simulink model "RC_3L_PWM"  (R2013b)
settings: Solver=FixedStepDiscrete  SolverMode=SingleTasking  StartTime=0.0  StopTime=1  FixedStep=Tpas  RelTol=1e-3
undefined symbols (not defined in the file): ASF3, Cbus, DAFE, fmod4Q, Freq, IAFE3L, Iv, Kac, Lac, NAFE, PAFE3L, Pv, Rac, Rch, Satv, Tpas, Vac, Vdc
libraries: powerlib x39, simulink x22, powerlib_meascontrol x16
settings Model: Creator=LiberT  LastModifiedBy=LiberT
settings DataIOCC: SignalLoggingSaveFormat=ModelDataLogs
settings OptimizationCC: ExpressionDepthLimit=2147483647
settings DebuggingCC: MultiTaskDSMMsg=warning  MultiTaskCondExecSysMsg=none  FcnCallInpInsideContextMsg=EnableAllAsWarning  StateNameClashWarn=warning
settings RTWCC: IncludeERTFirstTime=on

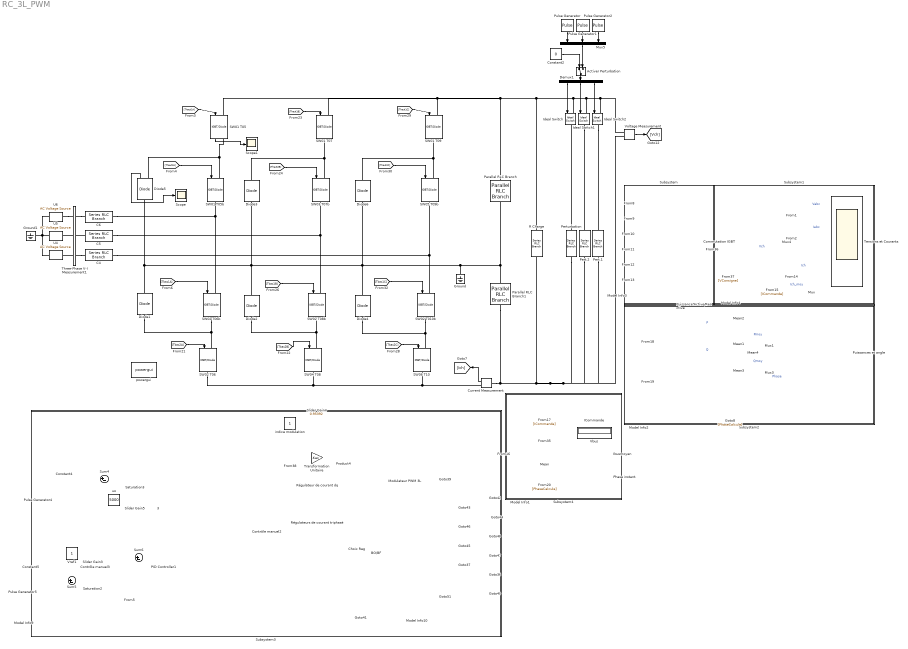
== system RC_3L_PWM ==
  " 3" : ManualSwitch
  Activer Perturbation : ManualSwitch
  BO/BF : ManualSwitch  CurrentSetting=0
  C4 : powerlib/Elements/Series RLC Branch  LConnTagsString=__new0  RConnTagsString=__new0  BranchType=L  Resistance=Rac  Inductance=Lac  SetiL0=off  InitialCurrent=0  Capacitance=300e-3  Setx0=off  InitialVoltage=0  Measurements=None
  C5 : powerlib/Elements/Series RLC Branch  LConnTagsString=__new0  RConnTagsString=__new0  BranchType=L  Resistance=Rac  Inductance=Lac  SetiL0=off  InitialCurrent=0  Capacitance=300e-3  Setx0=off  InitialVoltage=0  Measurements=None
  C6 : powerlib/Elements/Series RLC Branch  LConnTagsString=__new0  RConnTagsString=__new0  BranchType=L  Resistance=Rac  Inductance=Lac  SetiL0=off  InitialCurrent=0  Capacitance=300e-3  Setx0=off  InitialVoltage=0  Measurements=None
  Choix Reg : ManualSwitch  CurrentSetting=0
  Commutation IGBT : Scope  NumInputPorts=6
      settings: TickLabels=on  TimeRange=0.002  YMin=-0.2~-0.2~-0.2~-0.2~-0.2~-0.2  YMax=1.2~1.2~1.2~1.2~1.2~1.2
  Constant2 : Constant  Value=0
  Constant4 : Constant  Value=6000
  Constant5 : Constant  Value=6000
  Contrôle manuel2 : ManualSwitch  CurrentSetting=0
  Contrôle manuel3 : ManualSwitch
  Current Measurement : powerlib/Measurements/Current Measurement  PhasorSimulation=off  OutputType=Complex  PSBequivalent=0
  Demux1 : Demux  Outputs=3
  Diode{1..4,6} (5 alike) : powerlib/Power Electronics/Diode  Ron=0.001  Lon=0  Vf=0.8  IC=0  UseSnubber=off  Rs=500  Cs=inf  Measurements=off
  Diode5 : powerlib/Power Electronics/Diode  Ron=0.001  Lon=0  Vf=0.8  IC=0  UseSnubber=off  Rs=500  Cs=inf  Measurements=on
  Ground : powerlib/Elements/Ground  LConnTagsString=a
  Ground1 : powerlib/Elements/Ground  LConnTagsString=a
  "ICommande " : Display
  Ibusmoyen : Display
  Ideal Switch : powerlib/Power Electronics/Ideal Switch  Ron=0.001  Lon=0  IC=0  Rs=1e5  Cs=inf  Measurements=off
  Ideal Switch1 : powerlib/Power Electronics/Ideal Switch  Ron=0.001  Lon=0  IC=0  Rs=1e5  Cs=inf  Measurements=off
  Ideal Switch2 : powerlib/Power Electronics/Ideal Switch  Ron=0.001  Lon=0  IC=0  Rs=1e5  Cs=inf  Measurements=off
  Mean : powerlib_meascontrol/Measurements/Mean  Freq=50  Vinit=0  Ts=Tpas
  Mean1 : powerlib_meascontrol/Measurements/Mean  Freq=50  Vinit=0  Ts=Tpas
  Mean2 : powerlib_meascontrol/Measurements/Mean  Freq=fmod4Q  Vinit=0  Ts=Tpas
  Mean3 : powerlib_meascontrol/Measurements/Mean  Freq=50  Vinit=0  Ts=Tpas
  Mean4 : powerlib_meascontrol/Measurements/Mean  Freq=fmod4Q  Vinit=0  Ts=Tpas
  Model Info{1..4} (4 alike) : simulink/Model-Wide Utilities/Model Info  InitialBlockCM=None  BlockCM=None  Frame=on  DisplayStringWithTags=Résultats  HorizontalTextAlignment=Center  LeftAlignmentValue=0.5  SourceBlockDiagram=RC_3L_PWM  TagMaxNumber=20
  Model Info10 : simulink/Model-Wide Utilities/Model Info  InitialBlockCM=None  BlockCM=None  Frame=on  DisplayStringWithTags=Commande onduleur NPC3L  HorizontalTextAlignment=Center  LeftAlignmentValue=0.5  SourceBlockDiagram=RC_3L_PWM  TagMaxNumber=20
  Model Info9 : simulink/Model-Wide Utilities/Model Info  InitialBlockCM=None  BlockCM=None  Frame=on  DisplayStringWithTags=Commande AFE  HorizontalTextAlignment=Center  LeftAlignmentValue=0.5  SourceBlockDiagram=RC_3L_PWM  TagMaxNumber=20
  Modulateur PWM 3L : Subsystem
  Mux{,1,3..4} (4 alike) : Mux  Inputs=2
  Mux5 : Mux  Inputs=3
  PID Controller1 : simulink/Continuous/PID Controller  Controller=PI  TimeDomain=Discrete-time  SampleTime=Tpas  IntegratorMethod=Forward Euler  FilterMethod=Forward Euler  Form=Parallel  P=Pv  I=Iv  D=0  N=100  InitialConditionSource=internal  InitialConditionForIntegrator=0  InitialConditionForFilter=0  ExternalReset=none  LimitOutput=on  UpperSaturationLimit=Satv  LowerSaturationLimit=-Satv  LinearizeAsGain=on  AntiWindupMode=clamping  Kb=1  TrackingMode=off  Kt=1  PParamMin=[]  PParamMax=[]  IParamMin=[]  IParamMax=[]  DParamMin=[]  DParamMax=[]  NParamMin=[]  NParamMax=[]  KbParamMin=[]  KbParamMax=[]  KtParamMin=[]  KtParamMax=[]  POutMin=[]  POutMax=[]  IOutMin=[]  IOutMax=[]  DOutMin=[]  DOutMax=[]  NOutMin=[]  NOutMax=[]  KbOutMin=[]  KbOutMax=[]  KtOutMin=[]  KtOutMax=[]  IntegratorOutMin=[]  IntegratorOutMax=[]  FilterOutMin=[]  FilterOutMax=[]  SumOutMin=[]  SumOutMax=[]  SumI1OutMin=[]  SumI1OutMax=[]  SumI2OutMin=[]  SumI2OutMax=[]  SumI3OutMin=[]  SumI3OutMax=[]  SumDOutMin=[]  SumDOutMax=[]  SaturationOutMin=[]  SaturationOutMax=[]  IntegratorContinuousStateAttributes=''  IntegratorStateMustResolveToSignalObject=off  IntegratorRTWStateStorageClass=Auto  FilterContinuousStateAttributes=''  FilterStateMustResolveToSignalObject=off  FilterRTWStateStorageClass=Auto
  Parallel RLC Branch : powerlib/Elements/Parallel RLC Branch  LConnTagsString=a  RConnTagsString=__new0  BranchType=C  Resistance=9.26  Inductance=1e-3  SetiL0=off  InitialCurrent=0  Capacitance=Cbus*2  Setx0=on  InitialVoltage=Vdc/2  Measurements=None
  Parallel RLC Branch1 : powerlib/Elements/Parallel RLC Branch  LConnTagsString=a  RConnTagsString=__new0  BranchType=C  Resistance=9.26  Inductance=1e-3  SetiL0=off  InitialCurrent=0  Capacitance=Cbus*2  Setx0=on  InitialVoltage=Vdc/2  Measurements=None
  Pert.1 : powerlib/Elements/Series RLC Branch  LConnTagsString=__new0  RConnTagsString=__new0  BranchType=R  Resistance=50  Inductance=0  SetiL0=off  InitialCurrent=0  Capacitance=inf  Setx0=off  InitialVoltage=0  Measurements=None
  Pert.2 : powerlib/Elements/Series RLC Branch  LConnTagsString=__new0  RConnTagsString=__new0  BranchType=R  Resistance=50  Inductance=0  SetiL0=off  InitialCurrent=0  Capacitance=inf  Setx0=off  InitialVoltage=0  Measurements=None
  Perturbation : powerlib/Elements/Series RLC Branch  LConnTagsString=__new0  RConnTagsString=__new0  BranchType=R  Resistance=50  Inductance=0  SetiL0=off  InitialCurrent=0  Capacitance=inf  Setx0=off  InitialVoltage=0  Measurements=None
  Phase instant. : Display
  Product4 : Product
  Puissance Active/Reactive : Subsystem
  Puissances et angle : Scope  NumInputPorts=3
      settings: TickLabels=on  TimeRange=0.04  YMin=-5.5e+06~-500000~-120  YMax=500000~250000~50  SaveName=ScopeData2
  Pulse Generator : DiscretePulseGenerator  Period=floor((1/Tpas)/2)  PulseWidth=floor((1/Tpas)/4)  SampleTime=Tpas
  Pulse Generator1 : DiscretePulseGenerator  Period=floor((1/Tpas)/3)  PulseWidth=floor((1/Tpas)/6)  SampleTime=Tpas
  Pulse Generator2 : DiscretePulseGenerator  Period=floor((1/Tpas))  PulseWidth=floor((1/Tpas)/2)  SampleTime=Tpas
  Pulse Generator4 : DiscretePulseGenerator  Amplitude=12000  Period=floor(.4/Tpas)  PulseWidth=floor(.4/2/Tpas)  SampleTime=Tpas
  Pulse Generator5 : DiscretePulseGenerator  Amplitude=12000  Period=floor(.2/Tpas)  PulseWidth=floor(.2/2/Tpas)  SampleTime=Tpas
  R Charge : powerlib/Elements/Series RLC Branch  LConnTagsString=__new0  RConnTagsString=__new0  BranchType=R  Resistance=Rch  Inductance=0  SetiL0=off  InitialCurrent=0  Capacitance=inf  Setx0=off  InitialVoltage=0  Measurements=None
  Régulateur de courant dq : Subsystem
  Régulateurs de courant triphasé : Subsystem
  SW01 T05 : powerlib/Power Electronics/IGBT//Diode  Ron=1e-3  Rs=1e5  Cs=Tpas  Measurements=on
  SW01 T05b : powerlib/Power Electronics/IGBT//Diode  Ron=1e-3  Rs=1e5  Cs=Tpas  Measurements=off
  SW01 T07 : powerlib/Power Electronics/IGBT//Diode  Ron=1e-3  Rs=1e5  Cs=Tpas  Measurements=off
  SW01 T09 : powerlib/Power Electronics/IGBT//Diode  Ron=1e-3  Rs=1e5  Cs=Tpas  Measurements=off
  SW02 T010b : powerlib/Power Electronics/IGBT//Diode  Ron=1e-3  Rs=1e5  Cs=Tpas  Measurements=off
  SW02 T06 : powerlib/Power Electronics/IGBT//Diode  Ron=1e-3  Rs=1e5  Cs=Tpas  Measurements=off
  SW02 T06b : powerlib/Power Electronics/IGBT//Diode  Ron=1e-3  Rs=1e5  Cs=Tpas  Measurements=off
  SW02 T08b : powerlib/Power Electronics/IGBT//Diode  Ron=1e-3  Rs=1e5  Cs=Tpas  Measurements=off
  SW03 T07b : powerlib/Power Electronics/IGBT//Diode  Ron=1e-3  Rs=1e5  Cs=Tpas  Measurements=off
  SW04 T08 : powerlib/Power Electronics/IGBT//Diode  Ron=1e-3  Rs=1e5  Cs=Tpas  Measurements=off
  SW05 T09b : powerlib/Power Electronics/IGBT//Diode  Ron=1e-3  Rs=1e5  Cs=Tpas  Measurements=off
  SW06 T10 : powerlib/Power Electronics/IGBT//Diode  Ron=1e-3  Rs=1e5  Cs=Tpas  Measurements=off
  Saturation2 : Saturate  UpperLimit=5500  LowerLimit=4800
  Saturation3 : Saturate  UpperLimit=5000  LowerLimit=1000
  Scope : Scope
      settings: SaveName=DIODE
  Scope1 : Scope
      settings: SaveName=IGBT
  Slider Gain3 : simulink/Math Operations/Slider Gain  low=0  gain=5000  high=7000
  Slider Gain4 : simulink/Math Operations/Slider Gain  low=0  gain=0.95392  high=1
  Slider Gain5 : simulink/Math Operations/Slider Gain  low=0  gain=0  high=1
  Subsystem : Subsystem
      mask Display: disp('')
  Subsystem1 : Subsystem
      mask Display: disp('')
  Subsystem2 : Subsystem
      mask Display: disp('')
  Subsystem3 : Subsystem
      mask Display: disp('')
  Subsystem4 : Subsystem
      mask Display: disp('')
  Sum4 : Sum  Inputs=|+-
  Sum5 : Sum  Inputs=|+-
  Sum6 : Sum  Inputs=|+-
  Tensions et Courants : Scope  NumInputPorts=4
      settings: TickLabels=on  ShowLegends=on  TimeRange=0.4  YMin=-2000~-2000~5010~-2000  YMax=2000~2000~5100~2000  SaveName=AFE3LEVEL  MaxDataPoints=50000
  Three-Phase V-I Measurement1 : powerlib/Measurements/Three-Phase V-I Measurement  VoltageMeasurement=phase-to-ground  SetLabelV=on  LabelV=Vabc  Vpu=off  VpuLL=off  CurrentMeasurement=yes  SetLabelI=on  LabelI=Iabc  Ipu=off  Pbase=100e6  Vbase=500e3  OutputType=Complex  PhasorSimulation=off  PSBequivalent=0
  Transformation Unitaire : Gain  Gain=-Kac
  U4 : powerlib/Electrical Sources/AC Voltage Source  Amplitude=Vac*sqrt(2/3)  Phase=120  Frequency=Freq  SampleTime=Tpas  Measurements=Voltage
  U5 : powerlib/Electrical Sources/AC Voltage Source  Amplitude=Vac*sqrt(2/3)  Phase=-120  Frequency=Freq  SampleTime=Tpas  Measurements=Voltage
  U6 : powerlib/Electrical Sources/AC Voltage Source  Amplitude=Vac*sqrt(2/3)  Phase=0  Frequency=Freq  SampleTime=Tpas  Measurements=Voltage
  Vbus : Display
  Voltage Measurement : powerlib/Measurements/Voltage Measurement  PhasorSimulation=off  OutputType=Complex  PSBequivalent=0
  Vref1 : Constant  SampleTime=Tpas
  indice modulation : Constant
  powergui : powerlib/powergui  Priority=1  SimulationMode=Discrete  SolverType=Tustin  SampleTime=Tpas  frequency=60  SPID=off  DisableSnubberDevices=off  DisableRonSwitches=off  DisableVfSwitches=off  SwTol=0  Interpol=off  DisplayEquations=off  frequencyindice=50  Pbase=100e6  ErrMax=1e-4  Iterations=50  UnitsV=kV  UnitsW=MW  FunctionMessages=off  echomessages=off  HookPort=off  EnableUseOfTLC=off  x0status=blocks  RestoreLinks=warning  ResistiveCurrentMeasurement=off  Frange=[0:2:500]  Ylog=off  Xlog=on  ShowGrid=off  save=off  variable=ZData  structure=ScopeData  ZoomFFT=off  StartTime=0.25  cycles=4  DisplayStyle=1  fundamental=50  FreqAxis=off  MaxFrequency=5000  frequencyindicesteady=1  RmsSteady=1  display=off  Ts=0  methode=off
  uo : Constant  Value=5000
  wires:
  Current Measurement/1 -> [Ich]
  [T5] -> Commutation IGBT/1
  [T6] -> Commutation IGBT/2
  [T7] -> Commutation IGBT/3
  [T8] -> Commutation IGBT/4
  [T9] -> Commutation IGBT/5
  [T10] -> Commutation IGBT/6
  [Vabc] -> Tensions et Courants/1  "Vabc"
  [Iabc] -> Tensions et Courants/2  "Iabc"
  [Ich] -> Mux/1  "Ich"
  [ICommande] -> Mux/2  "Ich_moy"
  Mux/1 -> Tensions et Courants/4
  Mean/1 -> Ibusmoyen/1
  [Vch] -> Vbus/1
  [Ich] -> Mean/1
  [ICommande] -> "ICommande "/1
  [Vabc] -> Puissance Active/Reactive/1(Vabc)
  [Iabc] -> Puissance Active/Reactive/2(Iabc)
  Puissance Active/Reactive/1(P) -> Mean2/1, Mean1/1  "P"
  Puissance Active/Reactive/2(Q) -> Mean3/1, Mean4/1  "Q"
  Puissance Active/Reactive/3(PhC) -> Puissances et angle/3, [PhaseCalcule]  "Phase"
  Mean1/1 -> Mux1/2  "Pmoy"
  Mux1/1 -> Puissances et angle/1
  Mean3/1 -> Mux3/2  "Qmoy"
  Mux3/1 -> Puissances et angle/2
  Mux4/1 -> Tensions et Courants/3
  [Vch] -> Mux4/1  "Vch"
  Demux1/1 -> Ideal Switch/1
  Demux1/2 -> Ideal Switch1/1
  Demux1/3 -> Ideal Switch2/1
  Pulse Generator/1 -> Mux5/1
  Pulse Generator1/1 -> Mux5/2
  Pulse Generator2/1 -> Mux5/3
  Activer Perturbation/1 -> Demux1/1
  Mux5/1 -> Activer Perturbation/2
  [PhaseCalcule] -> Phase instant./1
  [Thaut1A] -> SW01 T05/1
  [Thaut2A] -> SW01 T05b/1
  [Tbas2A] -> SW02 T06/1
  [Thaut1B] -> SW01 T07/1
  [Thaut2B] -> SW03 T07b/1
  [Tbas2B] -> SW04 T08/1
  [Thaut1C] -> SW01 T09/1
  [Thaut2C] -> SW05 T09b/1
  [Tbas1C] -> SW02 T010b/1
  [Tbas2C] -> SW06 T10/1
  Voltage Measurement/1 -> [Vch]
  Constant2/1 -> Activer Perturbation/1
  [VConsigne] -> Mux4/2
  Mean2/1 -> Mux1/1
  Mean4/1 -> Mux3/1
  Diode5/1 -> Scope/1
  SW01 T05/1 -> Scope1/1
  Vref1/1 -> Slider Gain3/1
  Sum6/1 -> PID Controller1/1
  Contrôle manuel2/1 -> Régulateurs de courant triphasé/1(In1), Régulateur de courant dq/1(In1)
  Sum5/1 -> Saturation2/1
  Pulse Generator5/1 -> Sum5/1
  Constant5/1 -> Sum5/2
  Contrôle manuel3/1 -> Sum6/1
  Slider Gain3/1 -> Contrôle manuel3/1
  Saturation2/1 -> Contrôle manuel3/2
  Modulateur PWM 3L/1(Thaut1A) -> [Thaut1A]
  Modulateur PWM 3L/2(Thaut2A) -> [Thaut2A]
  Modulateur PWM 3L/3(Tbas1A) -> [Tbas1A]
  Modulateur PWM 3L/4(Tbas2A) -> [Tbas2A]
  Modulateur PWM 3L/5(Thaut1B) -> [Thaut1B]
  Modulateur PWM 3L/6(Thaut2B) -> [Thaut2B]
  Modulateur PWM 3L/7(Tbas1B) -> [Tbas1B]
  Modulateur PWM 3L/8(Tbas2B) -> [Tbas2B]
  Modulateur PWM 3L/9(Thaut1C) -> [Thaut1C]
  Modulateur PWM 3L/10(Thaut2C) -> [Thaut2C]
  Modulateur PWM 3L/11(Tbas1C) -> [Tbas1C]
  Modulateur PWM 3L/12(Tbas2C) -> [Tbas2C]
  indice modulation/1 -> Slider Gain4/1
  [Vabc] -> Transformation Unitaire/1
  Transformation Unitaire/1 -> Product4/2
  Slider Gain4/1 -> Product4/1
  BO/BF/1 -> Modulateur PWM 3L/1(Modulante3ph), [Modulante3ph]
  uo/1 -> Slider Gain5/1
  " 3"/1 -> Contrôle manuel2/1
  Slider Gain5/1 -> " 3"/2
  Saturation3/1 -> " 3"/1
  Sum4/1 -> Saturation3/1
  Pulse Generator4/1 -> Sum4/1
  Constant4/1 -> Sum4/2
  Choix Reg/1 -> BO/BF/2
  Régulateurs de courant triphasé/1(Sorties Régulateurs) -> Choix Reg/2
  Régulateur de courant dq/1(Sorties Régulateurs) -> Choix Reg/1
  Product4/1 -> BO/BF/1
  PID Controller1/1 -> Contrôle manuel2/2
  [Tbas1A] -> SW02 T06b/1
  [Tbas1B] -> SW02 T08b/1
  [Vch] -> Sum6/2
  connections:
  SW02 T06b/LConn1 -- SW01 T05b/RConn1 -- C6/LConn1
  SW02 T010b/LConn1 -- C4/LConn1 -- SW05 T09b/RConn1
  SW02 T08b/LConn1 -- C5/LConn1 -- SW03 T07b/RConn1
  Current Measurement/LConn1 -- Voltage Measurement/LConn2 -- Pert.1/RConn1 -- Pert.2/RConn1 -- Perturbation/RConn1 -- R Charge/RConn1 -- Parallel RLC Branch1/RConn1
  Ideal Switch1/RConn1 -- Pert.2/LConn1
  Ideal Switch2/RConn1 -- Pert.1/LConn1
  SW01 T05b/LConn1 -- Diode5/RConn1 -- SW01 T05/RConn1
  SW03 T07b/LConn1 -- Diode3/RConn1 -- SW01 T07/RConn1
  SW05 T09b/LConn1 -- Diode6/RConn1 -- SW01 T09/RConn1
  SW02 T06b/RConn1 -- Diode1/LConn1 -- SW02 T06/LConn1
  SW02 T010b/RConn1 -- Diode4/LConn1 -- SW06 T10/LConn1
  SW04 T08/LConn1 -- Diode2/LConn1 -- SW02 T08b/RConn1
  SW02 T06/RConn1 -- SW06 T10/RConn1 -- Current Measurement/RConn1 -- SW04 T08/RConn1
  SW01 T05/LConn1 -- SW01 T07/LConn1 -- SW01 T09/LConn1 -- Voltage Measurement/LConn1 -- Ideal Switch2/LConn1 -- Ideal Switch1/LConn1 -- Ideal Switch/LConn1 -- R Charge/LConn1 -- Parallel RLC Branch/LConn1
  Diode4/RConn1 -- Diode6/LConn1 -- Ground/LConn1 -- Parallel RLC Branch/RConn1 -- Parallel RLC Branch1/LConn1 -- Diode3/LConn1 -- Diode2/RConn1 -- Diode5/LConn1 -- Diode1/RConn1
  Three-Phase V-I Measurement1/RConn2 -- U5/RConn1
  Three-Phase V-I Measurement1/LConn1 -- C6/RConn1
  C5/RConn1 -- Three-Phase V-I Measurement1/LConn2
  Three-Phase V-I Measurement1/LConn3 -- C4/RConn1
  Three-Phase V-I Measurement1/RConn3 -- U4/RConn1
  U6/RConn1 -- Three-Phase V-I Measurement1/RConn1
  Ground1/LConn1 -- U4/LConn1 -- U6/LConn1 -- U5/LConn1
  Perturbation/LConn1 -- Ideal Switch/RConn1

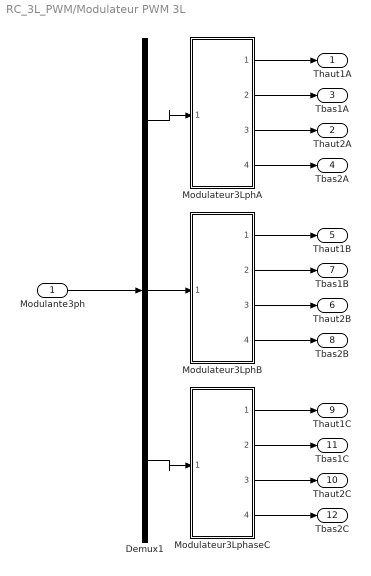
== system RC_3L_PWM/Modulateur PWM 3L ==
  Modulante3ph : Inport
  Demux1 : Demux  Outputs=3
  "Modulateur3LphA " : Subsystem
  Modulateur3LphB : Subsystem
  Modulateur3LphaseC : Subsystem
  Thaut1A : Outport
  Thaut2A : Outport  Port=2
  Tbas1A : Outport  Port=3
  Tbas2A : Outport  Port=4
  Thaut1B : Outport  Port=5
  Thaut2B : Outport  Port=6
  Tbas1B : Outport  Port=7
  Tbas2B : Outport  Port=8
  Thaut1C : Outport  Port=9
  Thaut2C : Outport  Port=10
  Tbas1C : Outport  Port=11
  Tbas2C : Outport  Port=12
  wires:
  Modulante3ph/1 -> Demux1/1
  Demux1/1 -> "Modulateur3LphA "/1(Modulante)
  "Modulateur3LphA "/1(Thaut1) -> Thaut1A/1
  "Modulateur3LphA "/2(Tbas1) -> Tbas1A/1
  "Modulateur3LphA "/3(Thaut2) -> Thaut2A/1
  "Modulateur3LphA "/4(Tbas2) -> Tbas2A/1
  Demux1/2 -> Modulateur3LphB/1(Modulante)
  Modulateur3LphB/1(Thaut1) -> Thaut1B/1
  Modulateur3LphB/2(Tbas1) -> Tbas1B/1
  Modulateur3LphB/3(Thaut2) -> Thaut2B/1
  Modulateur3LphB/4(Tbas2) -> Tbas2B/1
  Demux1/3 -> Modulateur3LphaseC/1(Modulante)
  Modulateur3LphaseC/1(Thaut1) -> Thaut1C/1
  Modulateur3LphaseC/2(Tbas1) -> Tbas1C/1
  Modulateur3LphaseC/3(Thaut2) -> Thaut2C/1
  Modulateur3LphaseC/4(Tbas2) -> Tbas2C/1

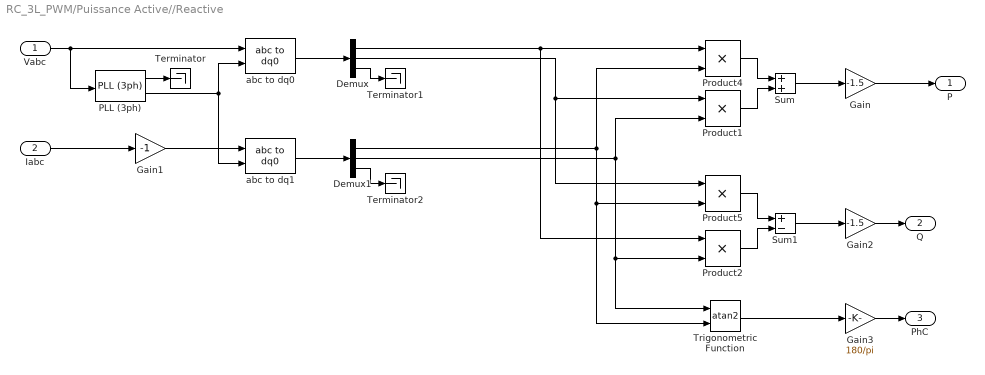
== system RC_3L_PWM/Puissance Active//Reactive ==
  Vabc : Inport
  Iabc : Inport  Port=2
  Demux : Demux  Outputs=3
  Demux1 : Demux  Outputs=3
  Gain : Gain  Gain=-1.5
  Gain1 : Gain  Gain=-1
  Gain2 : Gain  Gain=-1.5
  Gain3 : Gain  Gain=180/pi
  PLL (3ph) : powerlib_meascontrol/PLL/PLL (3ph)  Fmin=49  Par_Init=[0, 50]  ParK=[180, 3200, 1]  TcD=1e-4  MaxRateChangeFreq=6  FilterCutOffFreq=25  Ts=Tpas  AGC=on
  Product{1..2,4..5} (4 alike) : Product
  Sum : Sum
  Sum1 : Sum  Inputs=+-
  Terminator : Terminator
  Terminator1 : Terminator
  Terminator2 : Terminator
  Trigonometric Function : Trigonometry  Operator=atan2
  abc to dq0 : powerlib_meascontrol/Transformations/abc to dq0  Alignment=90 degrees behind phase A axis
  abc to dq1 : powerlib_meascontrol/Transformations/abc to dq0  Alignment=90 degrees behind phase A axis
  P : Outport
  Q : Outport  Port=2
  PhC : Outport  Port=3
  wires:
  Vabc/1 -> PLL (3ph)/1, abc to dq0/1
  abc to dq0/1 -> Demux/1
  abc to dq1/1 -> Demux1/1
  Product2/1 -> Sum1/2
  Sum1/1 -> Gain2/1
  Demux/2 -> Product5/1, Product1/1
  Demux/1 -> Product2/1, Product4/1
  Demux1/2 -> Trigonometric Function/1, Product2/2, Product1/2
  Product5/1 -> Sum1/1
  Gain2/1 -> Q/1
  Trigonometric Function/1 -> Gain3/1
  Gain3/1 -> PhC/1
  Product4/1 -> Sum/1
  Product1/1 -> Sum/2
  Sum/1 -> Gain/1
  Gain/1 -> P/1
  Demux1/1 -> Trigonometric Function/2, Product5/2, Product4/2
  PLL (3ph)/2 -> abc to dq1/2, abc to dq0/2
  Iabc/1 -> Gain1/1
  PLL (3ph)/1 -> Terminator/1
  Demux/3 -> Terminator1/1
  Demux1/3 -> Terminator2/1
  Gain1/1 -> abc to dq1/1

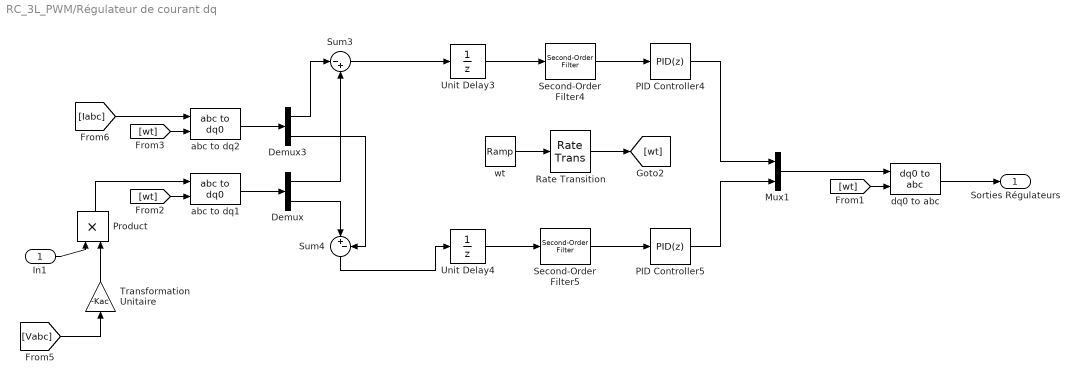
== system RC_3L_PWM/Régulateur de courant dq ==
  In1 : Inport
  Demux : Demux  Outputs=2
  Demux3 : Demux  Outputs=2
  Mux1 : Mux  Inputs=2
  PID Controller4 : simulink/Continuous/PID Controller  Controller=PID  TimeDomain=Discrete-time  SampleTime=Tpas  IntegratorMethod=Forward Euler  FilterMethod=Forward Euler  Form=Parallel  P=PAFE3L  I=IAFE3L  D=DAFE  N=NAFE  InitialConditionSource=internal  InitialConditionForIntegrator=0  InitialConditionForFilter=0  ExternalReset=none  LimitOutput=on  UpperSaturationLimit=0.95  LowerSaturationLimit=-0.95  LinearizeAsGain=on  AntiWindupMode=clamping  Kb=1  TrackingMode=off  Kt=1  PParamMin=[]  PParamMax=[]  IParamMin=[]  IParamMax=[]  DParamMin=[]  DParamMax=[]  NParamMin=[]  NParamMax=[]  KbParamMin=[]  KbParamMax=[]  KtParamMin=[]  KtParamMax=[]  POutMin=[]  POutMax=[]  IOutMin=[]  IOutMax=[]  DOutMin=[]  DOutMax=[]  NOutMin=[]  NOutMax=[]  KbOutMin=[]  KbOutMax=[]  KtOutMin=[]  KtOutMax=[]  IntegratorOutMin=[]  IntegratorOutMax=[]  FilterOutMin=[]  FilterOutMax=[]  SumOutMin=[]  SumOutMax=[]  SumI1OutMin=[]  SumI1OutMax=[]  SumI2OutMin=[]  SumI2OutMax=[]  SumI3OutMin=[]  SumI3OutMax=[]  SumDOutMin=[]  SumDOutMax=[]  SaturationOutMin=[]  SaturationOutMax=[]  IntegratorContinuousStateAttributes=''  IntegratorStateMustResolveToSignalObject=off  IntegratorRTWStateStorageClass=Auto  FilterContinuousStateAttributes=''  FilterStateMustResolveToSignalObject=off  FilterRTWStateStorageClass=Auto
  PID Controller5 : simulink/Continuous/PID Controller  Controller=PID  TimeDomain=Discrete-time  SampleTime=Tpas  IntegratorMethod=Forward Euler  FilterMethod=Forward Euler  Form=Parallel  P=PAFE3L  I=IAFE3L  D=DAFE  N=NAFE  InitialConditionSource=internal  InitialConditionForIntegrator=0  InitialConditionForFilter=0  ExternalReset=none  LimitOutput=on  UpperSaturationLimit=0.95  LowerSaturationLimit=-0.95  LinearizeAsGain=on  AntiWindupMode=clamping  Kb=1  TrackingMode=off  Kt=1  PParamMin=[]  PParamMax=[]  IParamMin=[]  IParamMax=[]  DParamMin=[]  DParamMax=[]  NParamMin=[]  NParamMax=[]  KbParamMin=[]  KbParamMax=[]  KtParamMin=[]  KtParamMax=[]  POutMin=[]  POutMax=[]  IOutMin=[]  IOutMax=[]  DOutMin=[]  DOutMax=[]  NOutMin=[]  NOutMax=[]  KbOutMin=[]  KbOutMax=[]  KtOutMin=[]  KtOutMax=[]  IntegratorOutMin=[]  IntegratorOutMax=[]  FilterOutMin=[]  FilterOutMax=[]  SumOutMin=[]  SumOutMax=[]  SumI1OutMin=[]  SumI1OutMax=[]  SumI2OutMin=[]  SumI2OutMax=[]  SumI3OutMin=[]  SumI3OutMax=[]  SumDOutMin=[]  SumDOutMax=[]  SaturationOutMin=[]  SaturationOutMax=[]  IntegratorContinuousStateAttributes=''  IntegratorStateMustResolveToSignalObject=off  IntegratorRTWStateStorageClass=Auto  FilterContinuousStateAttributes=''  FilterStateMustResolveToSignalObject=off  FilterRTWStateStorageClass=Auto
  Product : Product
  Rate Transition : RateTransition  OutPortSampleTime=Ts
  Second-Order Filter4 : powerlib_meascontrol/Filters/Second-Order Filter  FilterType=Lowpass  Fo=ASF3*fmod4Q  Zeta=QSF3  Ts=Tpas  Initialize=on  Vac_Init="[0,  0,  50]"  Vdc_Init=0  PlotResponse=off  FreqRange=[0, 10000, 1]
  Second-Order Filter5 : powerlib_meascontrol/Filters/Second-Order Filter  FilterType=Lowpass  Fo=ASF3*fmod4Q  Zeta=QSF3  Ts=Tpas  Initialize=on  Vac_Init="[0,  0,  50]"  Vdc_Init=0  PlotResponse=off  FreqRange=[0, 10000, 1]
  Sum3 : Sum  Inputs=|-+
  Sum4 : Sum  Inputs=|+-
  Transformation Unitaire : Gain  Gain=-Kac
  Unit Delay3 : UnitDelay  SampleTime=-1
  Unit Delay4 : UnitDelay  SampleTime=-1
  abc to dq1 : powerlib_meascontrol/Transformations/abc to dq0  Alignment=Aligned with phase A axis
  abc to dq2 : powerlib_meascontrol/Transformations/abc to dq0  Alignment=Aligned with phase A axis
  dq0 to abc : powerlib_meascontrol/Transformations/dq0 to abc  Alignment=Aligned with phase A axis
  wt : simulink/Sources/Ramp  slope=2*pi*50  start=0  X0=0
  Sorties Régulateurs : Outport
  wires:
  [Vabc] -> Transformation Unitaire/1
  Transformation Unitaire/1 -> Product/2
  In1/1 -> Product/1
  abc to dq1/1 -> Demux/1
  [wt] -> abc to dq1/2
  [wt] -> dq0 to abc/2
  wt/1 -> Rate Transition/1
  Rate Transition/1 -> [wt]
  Mux1/1 -> dq0 to abc/1
  Sum3/1 -> Unit Delay3/1
  PID Controller4/1 -> Mux1/1
  Demux/1 -> Sum3/2
  [Iabc] -> abc to dq2/1
  [wt] -> abc to dq2/2
  abc to dq2/1 -> Demux3/1
  Demux3/1 -> Sum3/1
  Product/1 -> abc to dq1/1
  Sum4/1 -> Unit Delay4/1
  PID Controller5/1 -> Mux1/2
  dq0 to abc/1 -> Sorties Régulateurs/1
  Unit Delay3/1 -> Second-Order Filter4/1
  Second-Order Filter4/1 -> PID Controller4/1
  Unit Delay4/1 -> Second-Order Filter5/1
  Second-Order Filter5/1 -> PID Controller5/1
  Demux/2 -> Sum4/1
  Demux3/2 -> Sum4/2

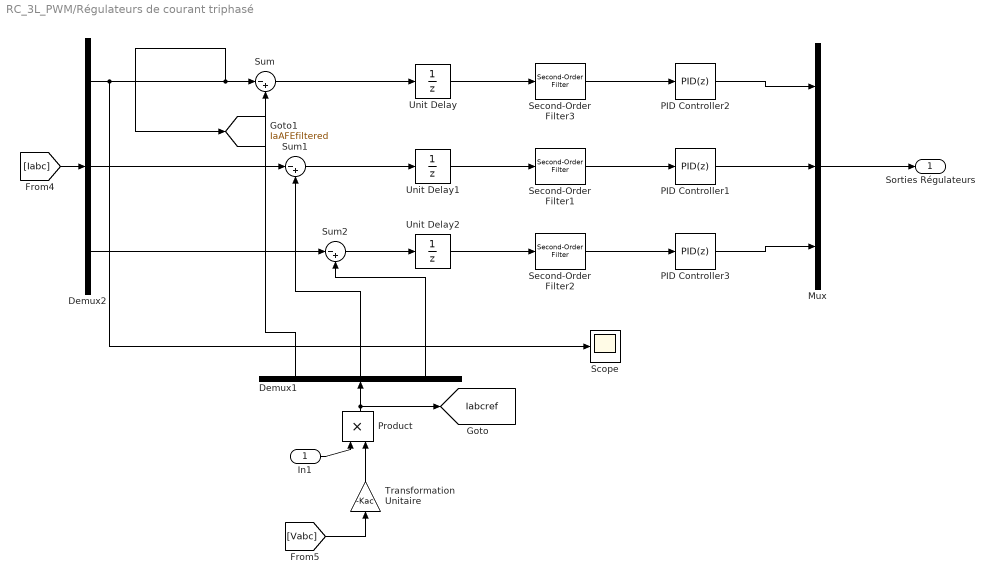
== system RC_3L_PWM/Régulateurs de courant triphasé ==
  In1 : Inport
  Demux1 : Demux  Outputs=3
  Demux2 : Demux  Outputs=3
  Mux : Mux  Inputs=3
  PID Controller1 : simulink/Continuous/PID Controller  Controller=PID  TimeDomain=Discrete-time  SampleTime=Tpas  IntegratorMethod=Forward Euler  FilterMethod=Forward Euler  Form=Parallel  P=PAFE3L  I=IAFE3L  D=DAFE  N=NAFE  InitialConditionSource=internal  InitialConditionForIntegrator=0  InitialConditionForFilter=0  ExternalReset=none  LimitOutput=on  UpperSaturationLimit=0.95  LowerSaturationLimit=-0.95  LinearizeAsGain=on  AntiWindupMode=clamping  Kb=1  TrackingMode=off  Kt=1  PParamMin=[]  PParamMax=[]  IParamMin=[]  IParamMax=[]  DParamMin=[]  DParamMax=[]  NParamMin=[]  NParamMax=[]  KbParamMin=[]  KbParamMax=[]  KtParamMin=[]  KtParamMax=[]  POutMin=[]  POutMax=[]  IOutMin=[]  IOutMax=[]  DOutMin=[]  DOutMax=[]  NOutMin=[]  NOutMax=[]  KbOutMin=[]  KbOutMax=[]  KtOutMin=[]  KtOutMax=[]  IntegratorOutMin=[]  IntegratorOutMax=[]  FilterOutMin=[]  FilterOutMax=[]  SumOutMin=[]  SumOutMax=[]  SumI1OutMin=[]  SumI1OutMax=[]  SumI2OutMin=[]  SumI2OutMax=[]  SumI3OutMin=[]  SumI3OutMax=[]  SumDOutMin=[]  SumDOutMax=[]  SaturationOutMin=[]  SaturationOutMax=[]  IntegratorContinuousStateAttributes=''  IntegratorStateMustResolveToSignalObject=off  IntegratorRTWStateStorageClass=Auto  FilterContinuousStateAttributes=''  FilterStateMustResolveToSignalObject=off  FilterRTWStateStorageClass=Auto
  PID Controller2 : simulink/Continuous/PID Controller  Controller=PID  TimeDomain=Discrete-time  SampleTime=Tpas  IntegratorMethod=Forward Euler  FilterMethod=Forward Euler  Form=Parallel  P=PAFE3L  I=IAFE3L  D=DAFE  N=NAFE  InitialConditionSource=internal  InitialConditionForIntegrator=0  InitialConditionForFilter=0  ExternalReset=none  LimitOutput=on  UpperSaturationLimit=0.95  LowerSaturationLimit=-0.95  LinearizeAsGain=on  AntiWindupMode=clamping  Kb=1  TrackingMode=off  Kt=1  PParamMin=[]  PParamMax=[]  IParamMin=[]  IParamMax=[]  DParamMin=[]  DParamMax=[]  NParamMin=[]  NParamMax=[]  KbParamMin=[]  KbParamMax=[]  KtParamMin=[]  KtParamMax=[]  POutMin=[]  POutMax=[]  IOutMin=[]  IOutMax=[]  DOutMin=[]  DOutMax=[]  NOutMin=[]  NOutMax=[]  KbOutMin=[]  KbOutMax=[]  KtOutMin=[]  KtOutMax=[]  IntegratorOutMin=[]  IntegratorOutMax=[]  FilterOutMin=[]  FilterOutMax=[]  SumOutMin=[]  SumOutMax=[]  SumI1OutMin=[]  SumI1OutMax=[]  SumI2OutMin=[]  SumI2OutMax=[]  SumI3OutMin=[]  SumI3OutMax=[]  SumDOutMin=[]  SumDOutMax=[]  SaturationOutMin=[]  SaturationOutMax=[]  IntegratorContinuousStateAttributes=''  IntegratorStateMustResolveToSignalObject=off  IntegratorRTWStateStorageClass=Auto  FilterContinuousStateAttributes=''  FilterStateMustResolveToSignalObject=off  FilterRTWStateStorageClass=Auto
  PID Controller3 : simulink/Continuous/PID Controller  Controller=PID  TimeDomain=Discrete-time  SampleTime=Tpas  IntegratorMethod=Forward Euler  FilterMethod=Forward Euler  Form=Parallel  P=PAFE3L  I=IAFE3L  D=DAFE  N=NAFE  InitialConditionSource=internal  InitialConditionForIntegrator=0  InitialConditionForFilter=0  ExternalReset=none  LimitOutput=on  UpperSaturationLimit=0.95  LowerSaturationLimit=-0.95  LinearizeAsGain=on  AntiWindupMode=clamping  Kb=1  TrackingMode=off  Kt=1  PParamMin=[]  PParamMax=[]  IParamMin=[]  IParamMax=[]  DParamMin=[]  DParamMax=[]  NParamMin=[]  NParamMax=[]  KbParamMin=[]  KbParamMax=[]  KtParamMin=[]  KtParamMax=[]  POutMin=[]  POutMax=[]  IOutMin=[]  IOutMax=[]  DOutMin=[]  DOutMax=[]  NOutMin=[]  NOutMax=[]  KbOutMin=[]  KbOutMax=[]  KtOutMin=[]  KtOutMax=[]  IntegratorOutMin=[]  IntegratorOutMax=[]  FilterOutMin=[]  FilterOutMax=[]  SumOutMin=[]  SumOutMax=[]  SumI1OutMin=[]  SumI1OutMax=[]  SumI2OutMin=[]  SumI2OutMax=[]  SumI3OutMin=[]  SumI3OutMax=[]  SumDOutMin=[]  SumDOutMax=[]  SaturationOutMin=[]  SaturationOutMax=[]  IntegratorContinuousStateAttributes=''  IntegratorStateMustResolveToSignalObject=off  IntegratorRTWStateStorageClass=Auto  FilterContinuousStateAttributes=''  FilterStateMustResolveToSignalObject=off  FilterRTWStateStorageClass=Auto
  Product : Product
  Scope : Scope
      settings: TimeRange=0.04  YMin=-6000  YMax=6000  SaveName=ScopeData2
  Second-Order Filter1 : powerlib_meascontrol/Filters/Second-Order Filter  FilterType=Lowpass  Fo=ASF3*fmod4Q  Zeta=QSF3  Ts=Tpas  Initialize=on  Vac_Init="[0,  0,  50]"  Vdc_Init=0  PlotResponse=off  FreqRange=[0, 10000, 1]
  Second-Order Filter2 : powerlib_meascontrol/Filters/Second-Order Filter  FilterType=Lowpass  Fo=ASF3*fmod4Q  Zeta=QSF3  Ts=Tpas  Initialize=on  Vac_Init="[0,  0,  50]"  Vdc_Init=0  PlotResponse=off  FreqRange=[0, 10000, 1]
  Second-Order Filter3 : powerlib_meascontrol/Filters/Second-Order Filter  FilterType=Lowpass  Fo=ASF3*fmod4Q  Zeta=QSF3  Ts=Tpas  Initialize=on  Vac_Init="[0,  0,  50]"  Vdc_Init=0  PlotResponse=off  FreqRange=[0, 10000, 1]
  Sum : Sum  Inputs=|-+
  Sum1 : Sum  Inputs=|-+
  Sum2 : Sum  Inputs=|-+
  Transformation Unitaire : Gain  Gain=-Kac
  Unit Delay : UnitDelay  SampleTime=-1
  Unit Delay1 : UnitDelay  SampleTime=-1
  Unit Delay2 : UnitDelay  SampleTime=-1
  Sorties Régulateurs : Outport
  tag scope: IaAFEfiltered=global, Iabcref=global
  wires:
  Sum/1 -> Unit Delay/1
  Sum1/1 -> Unit Delay1/1
  Sum2/1 -> Unit Delay2/1
  [Iabc] -> Demux2/1
  [Vabc] -> Transformation Unitaire/1
  Demux1/1 -> Sum/2
  Demux1/2 -> Sum1/2
  Demux1/3 -> Sum2/2
  Transformation Unitaire/1 -> Product/2
  In1/1 -> Product/1
  Product/1 -> Demux1/1, [Iabcref]
  PID Controller3/1 -> Mux/3
  PID Controller1/1 -> Mux/2
  PID Controller2/1 -> Mux/1
  Demux2/1 -> [IaAFEfiltered], Sum/1, Scope/1
  Demux2/2 -> Sum1/1
  Demux2/3 -> Sum2/1
  Second-Order Filter3/1 -> PID Controller2/1
  Unit Delay/1 -> Second-Order Filter3/1
  Unit Delay1/1 -> Second-Order Filter1/1
  Second-Order Filter1/1 -> PID Controller1/1
  Second-Order Filter2/1 -> PID Controller3/1
  Unit Delay2/1 -> Second-Order Filter2/1
  Mux/1 -> Sorties Régulateurs/1

== system RC_3L_PWM/Subsystem ==

== system RC_3L_PWM/Subsystem1 ==

== system RC_3L_PWM/Subsystem2 ==

== system RC_3L_PWM/Subsystem3 ==

== system RC_3L_PWM/Subsystem4 ==

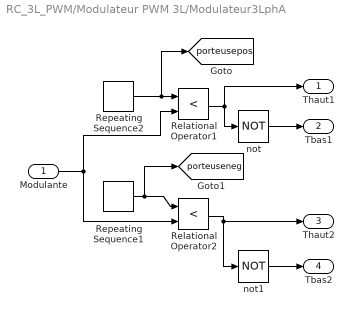
== system RC_3L_PWM/Modulateur PWM 3L/Modulateur3LphA  ==
  Modulante : Inport
  Relational Operator1 : RelationalOperator  Operator=<  OutDataTypeStr=boolean
  Relational Operator2 : RelationalOperator  Operator=<  OutDataTypeStr=boolean
  Repeating Sequence1 : simulink/Sources/Repeating Sequence  rep_seq_t=[0 .5/fmod4Q 1/fmod4Q]  rep_seq_y=[-1 0 -1]
  Repeating Sequence2 : simulink/Sources/Repeating Sequence  rep_seq_t=[0 .5/fmod4Q 1/fmod4Q]  rep_seq_y=[0 1 0]
  not : Logic  Operator=NOT  IconShape=distinctive  AllPortsSameDT=off  OutDataTypeStr=boolean
  not1 : Logic  Operator=NOT  IconShape=distinctive  AllPortsSameDT=off  OutDataTypeStr=boolean
  Thaut1 : Outport
  Tbas1 : Outport  Port=2
  Thaut2 : Outport  Port=3
  Tbas2 : Outport  Port=4
  tag scope: porteuseneg=global, porteusepos=global
  wires:
  Repeating Sequence2/1 -> [porteusepos], Relational Operator1/1
  Modulante/1 -> Relational Operator1/2, Relational Operator2/2
  Repeating Sequence1/1 -> [porteuseneg], Relational Operator2/1
  Relational Operator1/1 -> not/1, Thaut1/1
  not/1 -> Tbas1/1
  not1/1 -> Tbas2/1
  Relational Operator2/1 -> not1/1, Thaut2/1

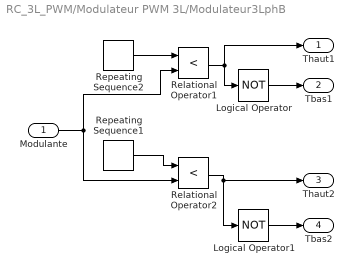
== system RC_3L_PWM/Modulateur PWM 3L/Modulateur3LphB ==
  Modulante : Inport
  Logical Operator : Logic  Operator=NOT  AllPortsSameDT=off  OutDataTypeStr=boolean
  Logical Operator1 : Logic  Operator=NOT  AllPortsSameDT=off  OutDataTypeStr=boolean
  Relational Operator1 : RelationalOperator  Operator=<  OutDataTypeStr=boolean
  Relational Operator2 : RelationalOperator  Operator=<  OutDataTypeStr=boolean
  Repeating Sequence1 : simulink/Sources/Repeating Sequence  rep_seq_t=[0 .5/fmod4Q 1/fmod4Q]  rep_seq_y=[-1 0 -1]
  Repeating Sequence2 : simulink/Sources/Repeating Sequence  rep_seq_t=[0 .5/fmod4Q 1/fmod4Q]  rep_seq_y=[0 1 0]
  Thaut1 : Outport
  Tbas1 : Outport  Port=2
  Thaut2 : Outport  Port=3
  Tbas2 : Outport  Port=4
  wires:
  Repeating Sequence2/1 -> Relational Operator1/1
  Modulante/1 -> Relational Operator1/2, Relational Operator2/2
  Repeating Sequence1/1 -> Relational Operator2/1
  Relational Operator1/1 -> Logical Operator/1, Thaut1/1
  Logical Operator/1 -> Tbas1/1
  Logical Operator1/1 -> Tbas2/1
  Relational Operator2/1 -> Logical Operator1/1, Thaut2/1

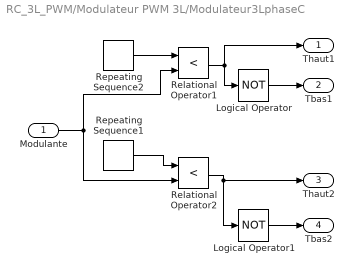
== system RC_3L_PWM/Modulateur PWM 3L/Modulateur3LphaseC ==
  Modulante : Inport
  Logical Operator : Logic  Operator=NOT  AllPortsSameDT=off  OutDataTypeStr=boolean
  Logical Operator1 : Logic  Operator=NOT  AllPortsSameDT=off  OutDataTypeStr=boolean
  Relational Operator1 : RelationalOperator  Operator=<  OutDataTypeStr=boolean
  Relational Operator2 : RelationalOperator  Operator=<  OutDataTypeStr=boolean
  Repeating Sequence1 : simulink/Sources/Repeating Sequence  rep_seq_t=[0 .5/fmod4Q 1/fmod4Q]  rep_seq_y=[-1 0 -1]
  Repeating Sequence2 : simulink/Sources/Repeating Sequence  rep_seq_t=[0 .5/fmod4Q 1/fmod4Q]  rep_seq_y=[0 1 0]
  Thaut1 : Outport
  Tbas1 : Outport  Port=2
  Thaut2 : Outport  Port=3
  Tbas2 : Outport  Port=4
  wires:
  Repeating Sequence2/1 -> Relational Operator1/1
  Modulante/1 -> Relational Operator1/2, Relational Operator2/2
  Repeating Sequence1/1 -> Relational Operator2/1
  Relational Operator1/1 -> Logical Operator/1, Thaut1/1
  Logical Operator/1 -> Tbas1/1
  Logical Operator1/1 -> Tbas2/1
  Relational Operator2/1 -> Logical Operator1/1, Thaut2/1
